simulink model "ejercicio1Comunicaciones"  (R2021a)
settings: Solver=VariableStepAuto  StartTime=0.0  StopTime=0.01  RelTol=1e-3
settings Model: SnapshotBufferSize=1  SnapshotInterval=1  Creator=jmata  LastModifiedBy=jmata

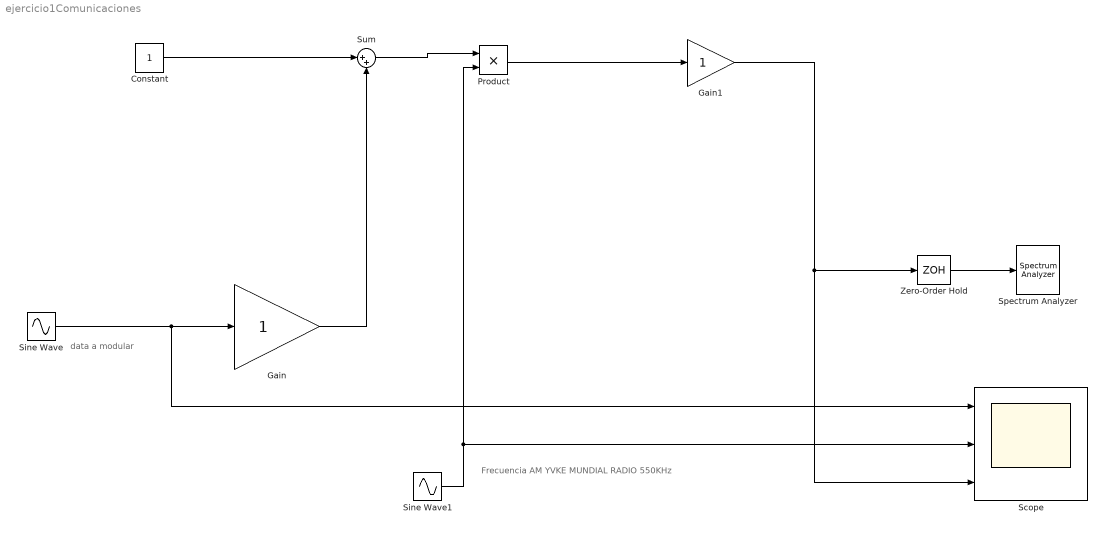
== system ejercicio1Comunicaciones ==
  note: Frecuencia AM YVKE MUNDIAL RADIO 550KHz
  note: data a modular
  Constant : Constant
  Gain : Gain
  Gain1 : Gain
  Product : Product
  Scope : Scope  NumInputPorts=3
  Sine Wave : Sin  Frequency=5e+3 * 2* pi  SampleTime=0
  Sine Wave1 : Sin  Frequency=550e+3 * 2 * pi  SampleTime=0
  Spectrum Analyzer : SpectrumAnalyzer
  Sum : Sum  Inputs=|++
  Zero-Order Hold : ZeroOrderHold  SampleTime=-1
  wires:
  Constant/1 -> Sum/1
  Gain/1 -> Sum/2
  Sine Wave/1 -> Scope/1, Gain/1
  Sine Wave1/1 -> Product/2, Scope/2
  Sum/1 -> Product/1
  Product/1 -> Gain1/1
  Gain1/1 -> Zero-Order Hold/1, Scope/3
  Zero-Order Hold/1 -> Spectrum Analyzer/1
